simulink model "Simulink_non_linear_3controls_model"  (R2016a)
settings: Solver=ode15s  SolverMode=SingleTasking  StartTime=0.0  StopTime=40  MaxStep=0.001  RelTol=1e-3
values from neighbouring files (symbols this model uses):
  TxBreak = 0    [setup.m]
  TxCoulomb = 2.5    [setup.m]
  TxVisc = 49.1750    (= 49.175)    [setup.m]
  TyBreak = 0    [setup.m]
  TyCoulomb = 1.8    [setup.m]
  TyVisc = 47.5650    (= 47.565)    [setup.m]
  TzVisc = 342    [setup.m]
undefined symbols (not defined in the file or in its folder): m, M, MR, sigbuilder_block, TzCoulomb
libraries: simulink x1
settings Model: Creator=Roy  LastModifiedBy=Roy
settings DebuggingCC: SFUnexpectedBacktrackingDiag=error  SFNoUnconditionalDefaultTransitionDiag=error
settings GRTTargetCC: TargetLangStandard=C99 (ISO)  GeneratePreprocessorConditionals=Use local settings
settings ConfigComp: CovMetricSettings=dwe  CovHtmlReporting=off  CovSaveCumulativeToWorkspaceVar=off  CovSaveSingleToWorkspaceVar=off  CovExternalEMLEnable=on

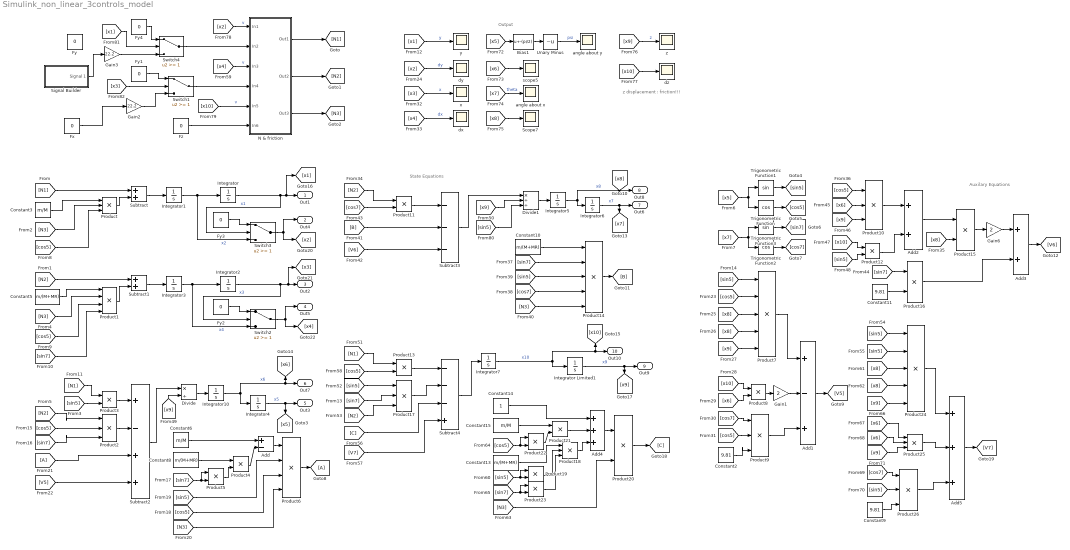
== system Simulink_non_linear_3controls_model ==
  note: Auxilary Equations
  note: State Equations
  note: Output
  note: z displacement : friction!!!
  Add : Sum  Inputs=+-
  Add1 : Sum  Inputs=+-+
  Add2 : Sum
  Add3 : Sum
  Add4 : Sum  Inputs=+++
  Add5 : Sum  Inputs=+++
  Bias1 : Bias  Bias=-(pi/2)
  Constant{5,8,10,13} (4 alike) : Constant  Value=m/(M+MR)
  Constant11 : Constant  Value=9.81
  Constant14 : Constant
  Constant15 : Constant  Value=m/M
  Constant2 : Constant  Value=9.81
  Constant3 : Constant  Value=m/M
  Constant6 : Constant  Value=m/M
  Constant9 : Constant  Value=9.81
  Divide : Product  Inputs=*/
  Divide1 : Product  Inputs=*//
  Fx : Constant  Value=0
  Fy{,1..4} (5 alike) : Constant  Value=0
  Fz : Constant  Value=0
  Gain1 : Gain  Gain=2
  Gain2 : Gain  Gain=22.2
  Gain3 : Gain  Gain=22.2
  Gain6 : Gain  Gain=2
  Integrator : Integrator  LimitOutput=on  UpperSaturationLimit=1  LowerSaturationLimit=0
  Integrator Limited1 : Integrator  InitialCondition=0.8  UpperSaturationLimit=-0.465  LowerSaturationLimit=-0.475
  Integrator{1,3,5..6,10} (5 alike) : Integrator
  Integrator2 : Integrator  LimitOutput=on  UpperSaturationLimit=1  LowerSaturationLimit=0
  Integrator4 : Integrator  InitialCondition=pi/2
  Integrator7 : Integrator  LimitOutput=on  UpperSaturationLimit=0.1  LowerSaturationLimit=-0.1
  N & friction : Subsystem
  Product{,2,9..10,17..18,25..26} (8 alike) : Product  Inputs=3
  Product1 : Product  Inputs=4
  Product{3..5,8,11..13,15..16,19..23} (14 alike) : Product
  Product14 : Product  Inputs=5
  Product24 : Product  Inputs=5
  Product6 : Product  Inputs=4
  Product7 : Product  Inputs=5
  Scope7 : Scope
  Signal Builder : Subsystem  Tag=STV Subsys  LoadFcn=sigbuilder_block('load');  StartFcn=sigbuilder_block('start');  StopFcn=sigbuilder_block('stop');  ClipboardFcn=sigbuilder_block('clipboard');  mask(Sigbuilder block){}
      mask help: Simulink:masks:SigbuilderBlock_MD
      mask init:
      | if ~strcmp(get_param(bdroot(gcbh),'SimulationStatus'),'stopped') tuvar = sigbuilder_block('maskInit'); end
      settings: CopyFcn=sigbuilder_block('copy');  DeleteFcn=sigbuilder_block('delete');  ModelCloseFcn=sigbuilder_block('modelClose');  PreSaveFcn=sigbuilder_block('preSave');  PauseFcn=sigbuilder_block('pause');  ContinueFcn=sigbuilder_block('continue');  NameChangeFcn=sigbuilder_block('namechange');  OpenFcn=sigbuilder_block('open',[437.6 199.2 550.4 400 ]);  CloseFcn=sigbuilder_block('close');
      mask Display: plot(0, 0, 100, 100,[2, 2, 32, 32, 2], [68, 8, 8, 68, 68],[32, 2], [38, 38], [32, 19, 2],[53, 60, 44], [32, 17, 17, 2],[16, 16, 31, 31]);txt = getActiveGroup(gcbh);text(2, 100, txt,'verticalAlignment', 'top');
  Subtract : Sum
  Subtract1 : Sum
  Subtract2 : Sum  Inputs=+-++
  Subtract3 : Sum  Inputs=---
  Subtract4 : Sum  Inputs=---+
  Switch{1..4} (4 alike) : Switch  Threshold=1
  Trigonometric Function : Trigonometry  Operator=cos
  Trigonometric Function1 : Trigonometry
  Trigonometric Function2 : Trigonometry  Operator=cos
  Trigonometric Function3 : Trigonometry
  Unary Minus : UnaryMinus
  angle about x : Scope
  angle about y : Scope
  dx : Scope
  dy : Scope
  dz : Scope
  scope5 : Scope
  x : Scope
  y : Scope
  z : Scope
  Out1 : Outport
  Out4 : Outport  Port=2
  Out2 : Outport  Port=3
  Out5 : Outport  Port=4
  Out3 : Outport  Port=5
  Out7 : Outport  Port=6
  Out6 : Outport  Port=7
  Out8 : Outport  Port=8
  Out9 : Outport  Port=9
  Out10 : Outport  Port=10
  wires:
  [N1] -> Subtract/1
  [N3] -> Product/2
  Constant3/1 -> Product/1
  Product/1 -> Subtract/2
  Subtract/1 -> Integrator1/1
  Integrator3/1 -> Integrator2/1, Switch2/3  "x4"
  Subtract1/1 -> Integrator3/1
  Product1/1 -> Subtract1/2
  Constant5/1 -> Product1/1
  [N3] -> Product1/2
  [N2] -> Subtract1/1
  Integrator2/1 -> Switch2/2, [x3], Out2/1  "x3"
  Integrator4/1 -> [x5], Out3/1  "x5"
  Product2/1 -> Subtract2/2
  [x5] -> Trigonometric Function/1, Trigonometric Function1/1
  [x7] -> Trigonometric Function3/1, Trigonometric Function2/1
  Trigonometric Function/1 -> [cos5]
  Trigonometric Function3/1 -> [sin7]
  Trigonometric Function2/1 -> [cos7]
  Trigonometric Function1/1 -> [sin5]
  [cos5] -> Product/3
  [cos5] -> Product1/3
  [sin7] -> Product1/4
  [N1] -> Product3/1
  [sin5] -> Product3/2
  Product3/1 -> Subtract2/1
  [N2] -> Product2/1
  [cos5] -> Product2/2
  [sin7] -> Product2/3
  Constant6/1 -> Add/1
  Constant8/1 -> Product4/1
  [sin7] -> Product5/1, Product5/2
  Product5/1 -> Product4/2
  Product4/1 -> Add/2
  Add/1 -> Product6/1
  [sin5] -> Product6/2
  [cos5] -> Product6/3
  [N3] -> Product6/4
  Product6/1 -> [A]
  [A] -> Subtract2/3
  [V5] -> Subtract2/4
  [sin5] -> Product7/1
  [cos5] -> Product7/2
  [x9] -> Product7/5
  [x8] -> Product7/4
  [x8] -> Product7/3
  Product7/1 -> Add1/1
  [x6] -> Product8/2
  [x10] -> Product8/1
  Gain1/1 -> Add1/2
  Product8/1 -> Gain1/1
  Product9/1 -> Add1/3
  [cos7] -> Product9/1
  [cos5] -> Product9/2
  Constant2/1 -> Product9/3
  Add1/1 -> [V5]
  Product14/1 -> [B]
  Product11/1 -> Subtract3/1
  [cos7] -> Product11/2
  [N2] -> Product11/1
  Integrator6/1 -> [x7], Out6/1  "x7"
  [B] -> Subtract3/2
  [V6] -> Subtract3/3
  Constant10/1 -> Product14/1
  [sin7] -> Product14/2
  [sin5] -> Product14/3
  [cos7] -> Product14/4
  [N3] -> Product14/5
  Product12/1 -> Add2/2
  [x10] -> Product12/1
  [sin5] -> Product12/2
  Product10/1 -> Add2/1
  [cos5] -> Product10/1
  [x6] -> Product10/2
  [x9] -> Product10/3
  Add3/1 -> [V6]
  Add2/1 -> Product15/1
  Product15/1 -> Gain6/1
  Gain6/1 -> Add3/1
  [x8] -> Product15/2
  [sin7] -> Product16/1
  Constant11/1 -> Product16/2
  Product16/1 -> Add3/2
  Subtract2/1 -> Divide/1
  Divide/1 -> Integrator10/1
  Subtract3/1 -> Divide1/1
  Divide1/1 -> Integrator5/1
  [x9] -> Divide1/2
  Integrator7/1 -> Out10/1, [x10], Integrator Limited1/1  "x10"
  [N1] -> Product13/1
  [cos5] -> Product13/2
  Product13/1 -> Subtract4/1
  Product20/1 -> [C]
  Add4/1 -> Product20/1
  Product19/1 -> Product18/2
  [sin5] -> Product19/2, Product19/1
  Constant13/1 -> Product18/1
  Product18/1 -> Add4/3
  Product21/1 -> Add4/2
  Constant14/1 -> Add4/1
  Constant15/1 -> Product21/1
  [cos5] -> Product22/1, Product22/2
  Product22/1 -> Product21/2
  [sin7] -> Product23/1, Product23/2
  [N3] -> Product20/2
  Product23/1 -> Product18/3
  [V7] -> Subtract4/4
  [C] -> Subtract4/3
  Product17/1 -> Subtract4/2
  [sin5] -> Product17/1
  [sin7] -> Product17/2
  [N2] -> Product17/3
  Add5/1 -> [V7]
  [sin5] -> Product26/2
  [cos7] -> Product26/1
  Product26/1 -> Add5/3
  Product25/1 -> Add5/2
  [x6] -> Product25/1
  [x6] -> Product25/2
  Product24/1 -> Add5/1
  [x8] -> Product24/3
  [x8] -> Product24/4
  [x9] -> Product24/5
  [sin5] -> Product24/2
  [sin5] -> Product24/1
  [x9] -> Product25/3
  Constant9/1 -> Product26/3
  [x1] -> y/1  "y"
  [x2] -> dy/1  "dy"
  [x3] -> x/1  "x"
  [x4] -> dx/1  "dx"
  [x8] -> Scope7/1
  [x7] -> angle about x/1  "theta"
  [x6] -> scope5/1
  [x9] -> z/1  "z"
  [x10] -> dz/1
  [x9] -> Divide/2
  Integrator10/1 -> [x6], Out7/1, Integrator4/1  "x6"
  Integrator5/1 -> [x8], Out8/1, Integrator6/1  "x8"
  Integrator Limited1/1 -> Out9/1, [x9]  "x9"
  [x2] -> N & friction/1(In1)  "v"
  [x4] -> N & friction/3(In3)  "v"
  [x10] -> N & friction/5(In5)  "v"
  Fz/1 -> N & friction/6(In6)
  N & friction/1(Out1) -> [N1]
  N & friction/2(Out2) -> [N2]
  N & friction/3(Out3) -> [N3]
  [sin5] -> Divide1/3
  Subtract4/1 -> Integrator7/1
  [x1] -> Switch4/2
  Fy4/1 -> Switch4/1
  Switch4/1 -> N & friction/2(In2)
  Fy1/1 -> Switch1/1
  [x3] -> Switch1/2
  Switch1/1 -> N & friction/4(In4)
  Fy3/1 -> Switch3/1
  Switch3/1 -> [x2], Out4/1
  Integrator1/1 -> Switch3/3, Integrator/1  "x2"
  Integrator/1 -> Switch3/2, [x1], Out1/1  "x1"
  Switch2/1 -> [x4], Out5/1
  Fy2/1 -> Switch2/1
  Gain2/1 -> Switch1/3
  Gain3/1 -> Switch4/3
  Unary Minus/1 -> angle about y/1  "psi"
  Bias1/1 -> Unary Minus/1
  [x5] -> Bias1/1
  Fx/1 -> Gain2/1
  Signal Builder/1(Signal 1) -> Gain3/1

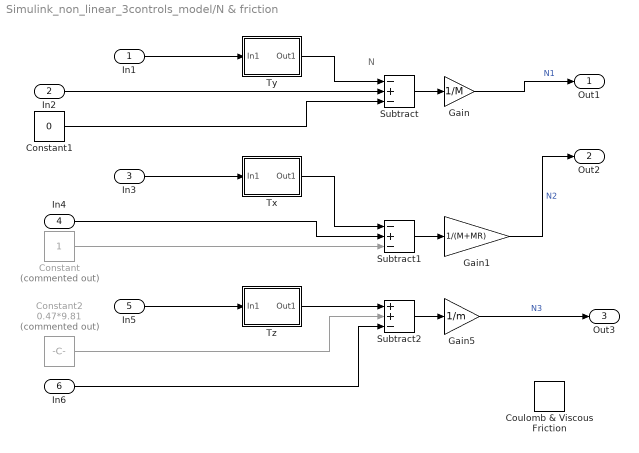
== system Simulink_non_linear_3controls_model/N & friction ==
  note: N
  In1 : Inport
  In2 : Inport  Port=2
  In3 : Inport  Port=3
  In4 : Inport  Port=4
  In5 : Inport  Port=5
  In6 : Inport  Port=6
  Constant : Constant  Commented=on
  Constant1 : Constant  Value=0
  Constant2 : Constant  Commented=on  Value=0.47*9.81
  Coulomb & Viscous Friction : simulink/Discontinuities/Coulomb & Viscous Friction  offset=[1 3 2 0]  gain=1
  Gain : Gain  Gain=1/M
  Gain1 : Gain  Gain=1/(M+MR)
  Gain5 : Gain  Gain=1/m
  Subtract : Sum  Inputs=-+-
  Subtract1 : Sum  Inputs=-+-
  Subtract2 : Sum  Inputs=++-
  Tx : Subsystem
  Ty : Subsystem
  Tz : Subsystem
  Out1 : Outport
  Out2 : Outport  Port=2
  Out3 : Outport  Port=3
  wires:
  In1/1 -> Ty/1(In1)
  In5/1 -> Tz/1(In1)
  In3/1 -> Tx/1(In1)
  Subtract1/1 -> Gain1/1
  Gain1/1 -> Out2/1  "N2"
  In2/1 -> Subtract/2
  In4/1 -> Subtract1/2
  Subtract/1 -> Gain/1
  Tx/1(Out1) -> Subtract1/1
  Ty/1(Out1) -> Subtract/1
  Tz/1(Out1) -> Subtract2/1
  Gain5/1 -> Out3/1  "N3"
  Subtract2/1 -> Gain5/1
  Gain/1 -> Out1/1  "N1"
  In6/1 -> Subtract2/3
  Constant/1 -> Subtract1/3
  Constant1/1 -> Subtract/3
  Constant2/1 -> Subtract2/2

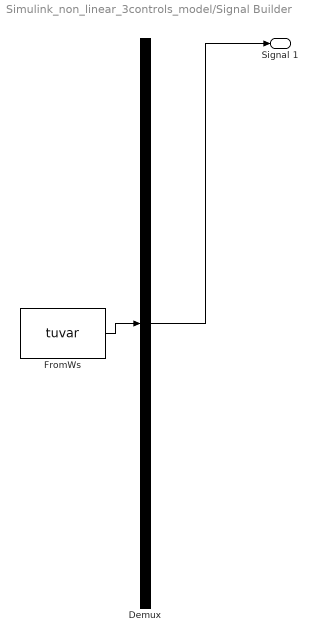
== system Simulink_non_linear_3controls_model/Signal Builder ==
  Demux : Demux  Tag=STV Demux  Outputs=1
  FromWs : FromWorkspace  Tag=STV FromWs  VariableName=tuvar  SampleTime=0
      SigBuilderData=|
      | common.afterFinalStr = 'Extrapolate'
      | common.sampleTime = 0
      | dataSet.timeRange = [0 10]
      | dataSet.name = 'Group 1'
      | sbobj.Groups.Name = 'Group 1'
      | sbobj.Groups.Signals.Name = 'Signal 1'
      | sbobj.Groups.Signals.XData = [0 1 1 2 2 10]
      | sbobj.Groups.Signals.YData = [0 0 0.8 0.8 0 0]
  Signal 1 : Outport  Tag=STV Outport
  wires:
  Demux/1 -> Signal 1/1
  FromWs/1 -> Demux/1

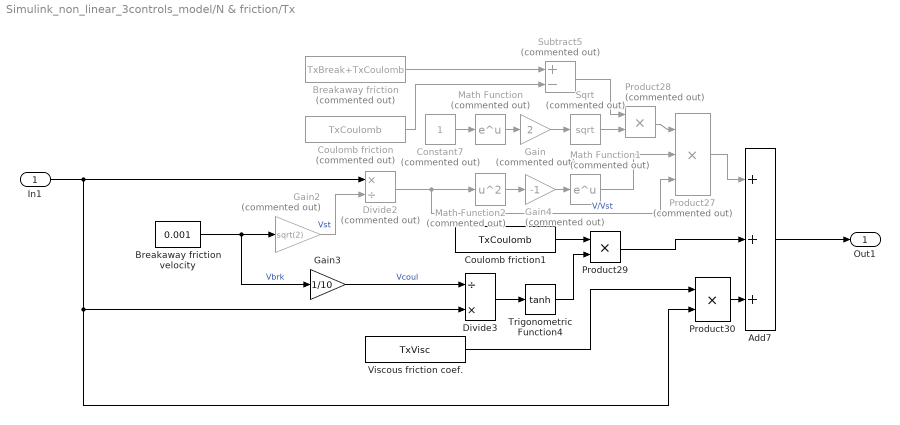
== system Simulink_non_linear_3controls_model/N & friction/Tx ==
  In1 : Inport
  Add7 : Sum  Inputs=+++
  Breakaway friction velocity : Constant  Value=0.001
  Breakaway friction : Constant  Commented=on  Value=TxBreak+TxCoulomb
  Constant7 : Constant  Commented=on
  Coulomb friction : Constant  Commented=on  Value=TxCoulomb
  Coulomb friction1 : Constant  Value=TxCoulomb
  Divide2 : Product  Commented=on  Inputs=*/
  Divide3 : Product  Inputs=/*
  Gain : Gain  Commented=on  Gain=2
  Gain2 : Gain  Commented=on  Gain=sqrt(2)
  Gain3 : Gain  Gain=1/10
  Gain4 : Gain  Commented=on  Gain=-1
  Math Function : Math  Commented=on  SaturateOnIntegerOverflow=on
  Math Function1 : Math  Commented=on  SaturateOnIntegerOverflow=on
  Math Function2 : Math  Commented=on  Operator=square  SaturateOnIntegerOverflow=on
  Product27 : Product  Commented=on  Inputs=3
  Product28 : Product  Commented=on
  Product29 : Product
  Product30 : Product
  Sqrt : Sqrt  Commented=on  SaturateOnIntegerOverflow=on
  Subtract5 : Sum  Commented=on  Inputs=+-
  Trigonometric Function4 : Trigonometry  Operator=tanh
  Viscous friction coef. : Constant  Value=TxVisc
  Out1 : Outport
  wires:
  Add7/1 -> Out1/1
  Divide2/1 -> Product27/3, Math Function2/1  "V/Vst"
  Product30/1 -> Add7/3
  Sqrt/1 -> Product28/2
  Product29/1 -> Add7/2
  Coulomb friction/1 -> Subtract5/2
  Subtract5/1 -> Product28/1
  Gain/1 -> Sqrt/1
  Product28/1 -> Product27/1
  Viscous friction coef./1 -> Product30/1
  Trigonometric Function4/1 -> Product29/2
  Breakaway friction/1 -> Subtract5/1
  Divide3/1 -> Trigonometric Function4/1
  Math Function/1 -> Gain/1
  Gain4/1 -> Math Function1/1
  Product27/1 -> Add7/1
  Breakaway friction velocity/1 -> Gain3/1, Gain2/1  "Vbrk"
  Math Function1/1 -> Product27/2
  Math Function2/1 -> Gain4/1
  Coulomb friction1/1 -> Product29/1
  Gain2/1 -> Divide2/2  "Vst"
  Constant7/1 -> Math Function/1
  In1/1 -> Divide3/2, Product30/2, Divide2/1
  Gain3/1 -> Divide3/1  "Vcoul"

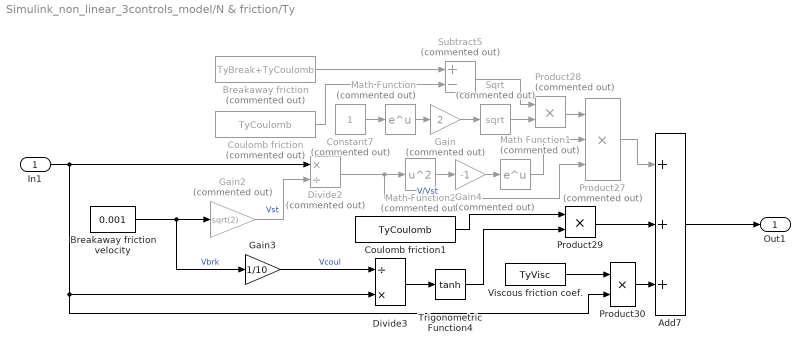
== system Simulink_non_linear_3controls_model/N & friction/Ty ==
  In1 : Inport
  Add7 : Sum  Inputs=+++
  Breakaway friction velocity : Constant  Value=0.001
  Breakaway friction : Constant  Commented=on  Value=TyBreak+TyCoulomb
  Constant7 : Constant  Commented=on
  Coulomb friction : Constant  Commented=on  Value=TyCoulomb
  Coulomb friction1 : Constant  Value=TyCoulomb
  Divide2 : Product  Commented=on  Inputs=*/
  Divide3 : Product  Inputs=/*
  Gain : Gain  Commented=on  Gain=2
  Gain2 : Gain  Commented=on  Gain=sqrt(2)
  Gain3 : Gain  Gain=1/10
  Gain4 : Gain  Commented=on  Gain=-1
  Math Function : Math  Commented=on  SaturateOnIntegerOverflow=on
  Math Function1 : Math  Commented=on  SaturateOnIntegerOverflow=on
  Math Function2 : Math  Commented=on  Operator=square  SaturateOnIntegerOverflow=on
  Product27 : Product  Commented=on  Inputs=3
  Product28 : Product  Commented=on
  Product29 : Product
  Product30 : Product
  Sqrt : Sqrt  Commented=on  SaturateOnIntegerOverflow=on
  Subtract5 : Sum  Commented=on  Inputs=+-
  Trigonometric Function4 : Trigonometry  Operator=tanh
  Viscous friction coef. : Constant  Value=TyVisc
  Out1 : Outport
  wires:
  Gain3/1 -> Divide3/1  "Vcoul"
  In1/1 -> Divide2/1, Product30/2, Divide3/2
  Constant7/1 -> Math Function/1
  Gain2/1 -> Divide2/2  "Vst"
  Coulomb friction1/1 -> Product29/1
  Math Function2/1 -> Gain4/1
  Math Function1/1 -> Product27/2
  Breakaway friction velocity/1 -> Gain2/1, Gain3/1  "Vbrk"
  Product27/1 -> Add7/1
  Gain4/1 -> Math Function1/1
  Math Function/1 -> Gain/1
  Divide3/1 -> Trigonometric Function4/1
  Breakaway friction/1 -> Subtract5/1
  Trigonometric Function4/1 -> Product29/2
  Viscous friction coef./1 -> Product30/1
  Product28/1 -> Product27/1
  Gain/1 -> Sqrt/1
  Subtract5/1 -> Product28/1
  Coulomb friction/1 -> Subtract5/2
  Product29/1 -> Add7/2
  Sqrt/1 -> Product28/2
  Product30/1 -> Add7/3
  Divide2/1 -> Math Function2/1, Product27/3  "V/Vst"
  Add7/1 -> Out1/1

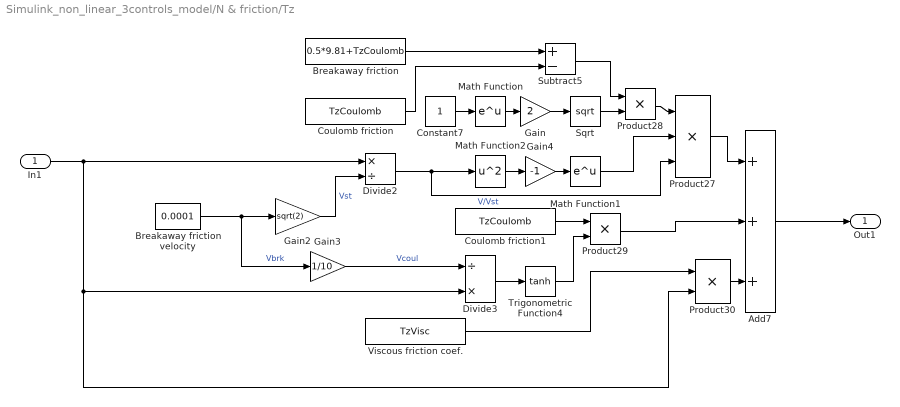
== system Simulink_non_linear_3controls_model/N & friction/Tz ==
  In1 : Inport
  Add7 : Sum  Inputs=+++
  Breakaway friction velocity : Constant  Value=0.0001
  Breakaway friction : Constant  Value=0.5*9.81+TzCoulomb
  Constant7 : Constant
  Coulomb friction : Constant  Value=TzCoulomb
  Coulomb friction1 : Constant  Value=TzCoulomb
  Divide2 : Product  Inputs=*/
  Divide3 : Product  Inputs=/*
  Gain : Gain  Gain=2
  Gain2 : Gain  Gain=sqrt(2)
  Gain3 : Gain  Gain=1/10
  Gain4 : Gain  Gain=-1
  Math Function : Math  SaturateOnIntegerOverflow=on
  Math Function1 : Math  SaturateOnIntegerOverflow=on
  Math Function2 : Math  Operator=square  SaturateOnIntegerOverflow=on
  Product27 : Product  Inputs=3
  Product28 : Product
  Product29 : Product
  Product30 : Product
  Sqrt : Sqrt  SaturateOnIntegerOverflow=on
  Subtract5 : Sum  Inputs=+-
  Trigonometric Function4 : Trigonometry  Operator=tanh
  Viscous friction coef. : Constant  Value=TzVisc
  Out1 : Outport
  wires:
  Gain3/1 -> Divide3/1  "Vcoul"
  In1/1 -> Divide2/1, Product30/2, Divide3/2
  Constant7/1 -> Math Function/1
  Gain2/1 -> Divide2/2  "Vst"
  Coulomb friction1/1 -> Product29/1
  Math Function2/1 -> Gain4/1
  Math Function1/1 -> Product27/2
  Breakaway friction velocity/1 -> Gain2/1, Gain3/1  "Vbrk"
  Product27/1 -> Add7/1
  Gain4/1 -> Math Function1/1
  Math Function/1 -> Gain/1
  Divide3/1 -> Trigonometric Function4/1
  Breakaway friction/1 -> Subtract5/1
  Trigonometric Function4/1 -> Product29/2
  Viscous friction coef./1 -> Product30/1
  Product28/1 -> Product27/1
  Gain/1 -> Sqrt/1
  Subtract5/1 -> Product28/1
  Coulomb friction/1 -> Subtract5/2
  Product29/1 -> Add7/2
  Sqrt/1 -> Product28/2
  Product30/1 -> Add7/3
  Divide2/1 -> Math Function2/1, Product27/3  "V/Vst"
  Add7/1 -> Out1/1
